simulink model "combined"  (R2023a)
settings: Solver=FixedStepAuto  StartTime=0.0  StopTime=30  RelTol=1e-3
values from neighbouring files (symbols this model uses):
  vehicle_data = getVehicleDataStruct()    [main.m]
libraries: autolibshared x4
settings Model: Creator=ashkan  LastModifiedBy=ashkan
settings OptimizationCC: ReuseModelBlockBuffer=off

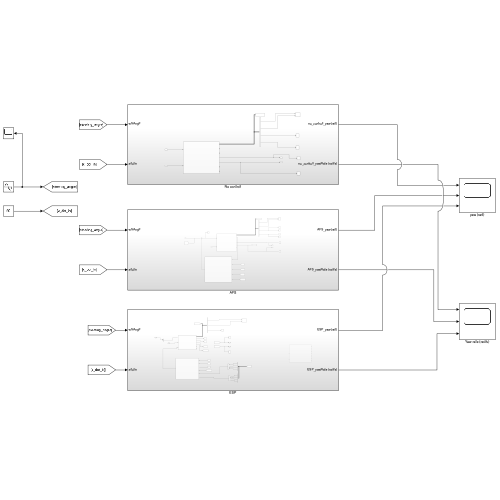
[thumbnail: Simulink's stored preview of the top-level diagram]
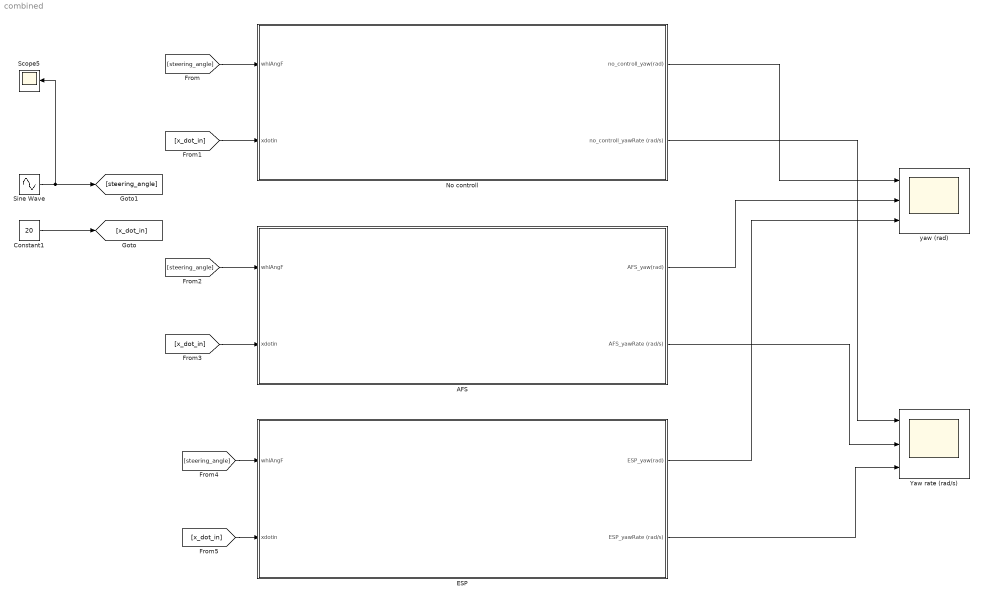
== system combined ==
  AFS : Subsystem
  Constant1 : Constant  Value=20
  ESP : Subsystem
  No controll : Subsystem
  Scope5 : Scope
  Sine Wave : Sin  Amplitude=2  Frequency=0.5  SampleTime=0
  Yaw rate (rad/s) : Scope  NumInputPorts=3
  yaw (rad) : Scope  NumInputPorts=3
  wires:
  Sine Wave/1 -> [steering_angle], Scope5/1
  Constant1/1 -> [x_dot_in]
  [steering_angle] -> No controll/1(whlAngF)
  [x_dot_in] -> No controll/2(xdotin)
  [steering_angle] -> AFS/1(whlAngF)
  [x_dot_in] -> AFS/2(xdotin)
  [steering_angle] -> ESP/1(whlAngF)
  [x_dot_in] -> ESP/2(xdotin)
  No controll/1(no_controll_yaw(rad)) -> yaw (rad)/1
  AFS/1(AFS_yaw(rad)) -> yaw (rad)/2
  ESP/1(ESP_yaw(rad)) -> yaw (rad)/3
  No controll/2(no_controll_yawRate (rad/s)) -> Yaw rate (rad/s)/1
  AFS/2(AFS_yawRate (rad/s)) -> Yaw rate (rad/s)/2
  ESP/2(ESP_yawRate (rad/s)) -> Yaw rate (rad/s)/3

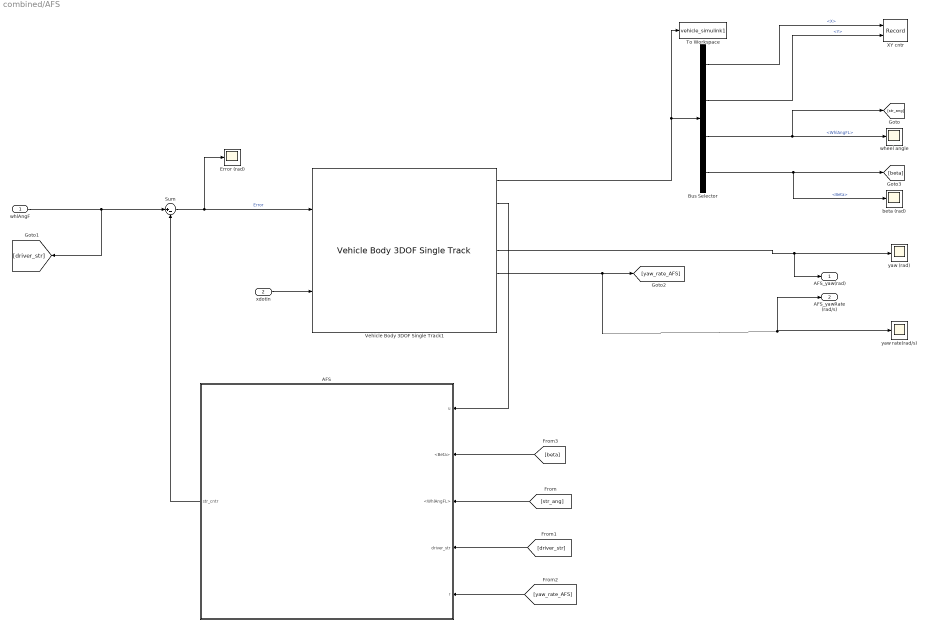
== system combined/AFS ==
  whlAngF : Inport
  xdotin : Inport  Port=2
  AFS : Subsystem
  Bus Selector : BusSelector  OutputSignals=InertFrm.Cg.Disp.X,InertFrm.Cg.Disp.Y,BdyFrm.FrntAxl.Steer.WhlAngFL,BdyFrm.Cg.Ang.Beta
  Error (rad) : Scope
  Sum : Sum  Inputs=|+-
  To Workspace : ToWorkspace  VariableName=vehicle_simulink1  SaveFormat=Timeseries  SampleTime=-1
  Vehicle Body 3DOF Single Track1 : autolibshared/Vehicle Body 3DOF Single Track  trackMode=Single (bicycle)  inputMode=External longitudinal velocity  frontSteerMode=on  rearSteerMode=off  windMode=off  muMode=off  extFMode=off  extMMode=off  htchFMode=off  htchMMode=off  extXo=off  extpsio=off  extxdoto=off  extro=off  extYo=off  extTamb=off  extydoto=off  aMode=2  NF=2  NR=2  m=vehicle_data.vehicle.m  a=vehicle_data.vehicle.Lf  b=vehicle_data.vehicle.Lr  h=vehicle_data.vehicle.hGs  dh=1  hh=0.2  X_o=0  xdot_o=0  CalphaMode=off  sigmaMode=on  d=0  hl=0  w=[1.4,1.4]  Cy_f=vehicle_data.front_suspension.Ks_f  Cy_r=vehicle_data.rear_suspension.Ks_r  sigma_f=.1  sigma_r=.1  alpha_f_brk=[-.1 .1]  Cy_f_data=[-9e3 9e3]  alpha_r_brk=[-.1 .1]  Cy_r_data=[-9e3 9e3]  Y_o=0  ydot_o=0  Izz=vehicle_data.vehicle.i_zz  psi_o=0  r_o=0  Af=2  Cd=.3  Cl=.1  Cpm=.1  beta_w=[0 0.01:0.01:0.3]  Cs=[0 0.01:0.01:0.3]  Cym=[0 1e-6:0.01:0.3]  Pabs=101325  Tair=273  g=9.81  mu=1  xdot_tol=.01  Fznom=5000  Fxtire_sat=7e4  Fytire_sat=7e4  longOff=0  latOff=0  vertOff=0  wrapAng=off
  XY cntr : Record  FileSettingsInternal="{\"entries\":[{\"content\":{\"excelSettings\":{\"content\":{},\"type\":\"Streamout.ExcelSettings\"}},\"type\":\"Streamout.FileSettingStorage\",\"uuid\":\"\"}],\"packageUris\":[\"http:\\/\\/schema.mathworks.com\\/mf0\\/streamout_blocks\\/R2020a\"],\"version\":\"1.0\"}"  Layout=[1 1]  SignalsInternal="{\"entries\":[{\"content\":{\"signals\":[{\"content\":{\"blockPath\":[],\"dimensions\":[1],\"domain\":\"\",\"lineColor\":\"#77ac30\",\"port\":1,\"sid\":[\"\"],\"signalID\":275,\"signalName\":\"<X>\"},\"type\":\"RecordBlkView.Signal\",\"uuid\":\"\"},{\"content\":{\"blockPath\":[],\"dimensions\":[1],\"domain\":\"\",\"lineColor\":\"#4dbeee\",\"port\":2,\"sid\":[\"\"],\"signalID\":279,\"signalName\":\"<Y>\"},\"type\":\"RecordBlkView.Signal\",\"uuid\":\"\"}]},\"type\":\"RecordBlkView.InputSignals\",\"uuid\":\"\"}],\"packageUris\":[\"http:\\/\\/schema.mathworks.com\\/mf0\\/streamout_blocks\\/R2020a\"],\"version\":\"1.0\"}"  VisualizationBindings="{\"xyplotplugin\":{\"info\":[{\"series\":[],\"subplotID\":1}]}}"  CompatibilityTag=XY
  beta (rad) : Scope
  wheel angle : Scope
  yaw (rad) : Scope
  yaw rate(rad/s) : Scope
  AFS_yaw(rad) : Outport
  AFS_yawRate (rad/s) : Outport  Port=2
  wires:
  whlAngF/1 -> [driver_str], Sum/1
  Sum/1 -> Error (rad)/1, Vehicle Body 3DOF Single Track1/1  "Error"
  [yaw_rate_AFS] -> AFS/5(r)
  Bus Selector/3 -> [str_ang], wheel angle/1  "<WhlAngFL>"
  Bus Selector/2 -> XY cntr/2  "<Y>"
  Vehicle Body 3DOF Single Track1/1 -> To Workspace/1, Bus Selector/1
  [beta] -> AFS/2(<Beta>)
  Bus Selector/1 -> XY cntr/1  "<X>"
  Bus Selector/4 -> [beta], beta (rad)/1  "<Beta>"
  AFS/1(str_cntr) -> Sum/2
  Vehicle Body 3DOF Single Track1/2 -> AFS/1(u)
  xdotin/1 -> Vehicle Body 3DOF Single Track1/2
  Vehicle Body 3DOF Single Track1/5 -> [yaw_rate_AFS], AFS_yawRate (rad/s)/1, yaw rate(rad/s)/1
  Vehicle Body 3DOF Single Track1/4 -> AFS_yaw(rad)/1, yaw (rad)/1
  [str_ang] -> AFS/3(<WhlAngFL>)
  [driver_str] -> AFS/4(driver_str)

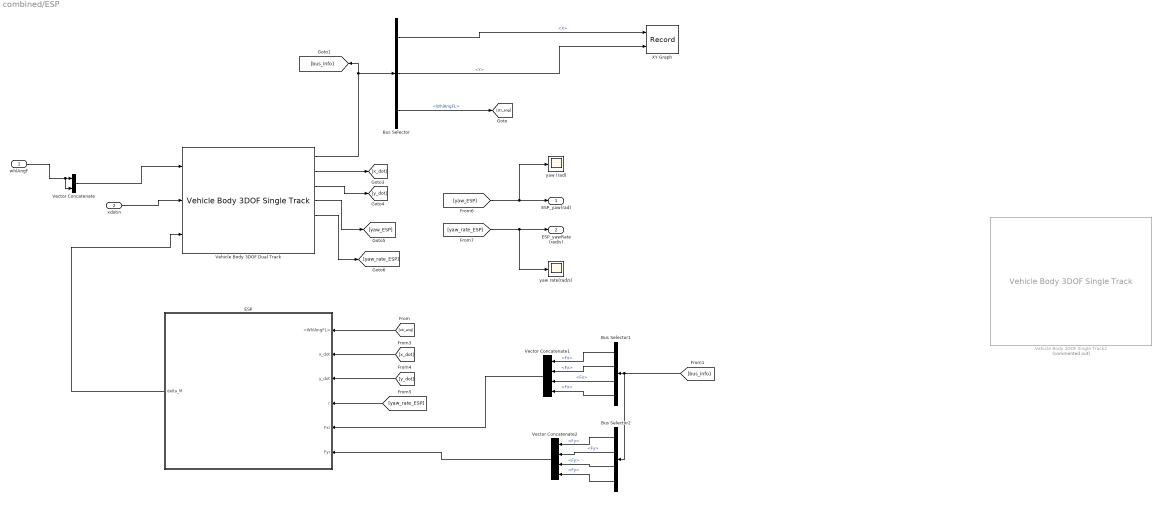
== system combined/ESP ==
  whlAngF : Inport
  xdotin : Inport  Port=2
  Bus Selector : BusSelector  OutputSignals=InertFrm.Cg.Disp.X,InertFrm.Cg.Disp.Y,BdyFrm.FrntAxl.Steer.WhlAngFL
  Bus Selector1 : BusSelector  OutputSignals=BdyFrm.Forces.FrntAxl.Lft.Fx,BdyFrm.Forces.RearAxl.Rght.Fx,BdyFrm.Forces.RearAxl.Lft.Fx,BdyFrm.Forces.FrntAxl.Rght.Fx
  Bus Selector2 : BusSelector  OutputSignals=BdyFrm.Forces.FrntAxl.Lft.Fy,BdyFrm.Forces.FrntAxl.Rght.Fy,BdyFrm.Forces.RearAxl.Lft.Fy,BdyFrm.Forces.RearAxl.Rght.Fy
  ESP : Subsystem
  Vector Concatenate : Concatenate
  Vector Concatenate1 : Concatenate  NumInputs=4
  Vector Concatenate2 : Concatenate  NumInputs=4
  Vehicle Body 3DOF Dual Track : autolibshared/Vehicle Body 3DOF Single Track  trackMode=Dual  inputMode=External longitudinal velocity  frontSteerMode=on  rearSteerMode=off  windMode=off  muMode=off  extFMode=off  extMMode=on  htchFMode=off  htchMMode=off  extXo=off  extpsio=off  extxdoto=off  extro=off  extYo=off  extTamb=off  extydoto=off  aMode=2  NF=2  NR=2  m=2000  a=1.4  b=1.6  h=0.35  dh=1  hh=0.2  X_o=0  xdot_o=0  CalphaMode=off  sigmaMode=on  d=0  hl=0  w=[1.4,1.4]  Cy_f=12e3  Cy_r=11e3  sigma_f=.1  sigma_r=.1  alpha_f_brk=[-.1 .1]  Cy_f_data=[-9e3 9e3]  alpha_r_brk=[-.1 .1]  Cy_r_data=[-9e3 9e3]  Y_o=0  ydot_o=0  Izz=4000  psi_o=0  r_o=0  Af=2  Cd=.3  Cl=.1  Cpm=.1  beta_w=[0 0.01:0.01:0.3]  Cs=[0:0.03:0.9]  Cym=[0 1e-6:0.01:0.3]  Pabs=101325  Tair=273  g=9.81  mu=1  xdot_tol=.01  Fznom=5000  Fxtire_sat=7e4  Fytire_sat=7e4  longOff=0  latOff=0  vertOff=0  wrapAng=off
      settings: LibrarySourceBlock=vehdynlibeom/Vehicle Body 3DOF Dual Track
  Vehicle Body 3DOF Single Track2 : autolibshared/Vehicle Body 3DOF Single Track  Commented=on  trackMode=Dual  inputMode=External longitudinal velocity  frontSteerMode=on  rearSteerMode=off  windMode=off  muMode=off  extFMode=off  extMMode=on  htchFMode=off  htchMMode=off  extXo=off  extpsio=off  extxdoto=off  extro=off  extYo=off  extTamb=off  extydoto=off  aMode=2  NF=2  NR=2  m=vehicle_data.vehicle.m  a=vehicle_data.vehicle.Lf  b=vehicle_data.vehicle.Lr  h=vehicle_data.vehicle.hGs  dh=1  hh=0.2  X_o=0  xdot_o=0  CalphaMode=off  sigmaMode=on  d=0  hl=0  w=[vehicle_data.vehicle.Wf,vehicle_data.vehicle.Wr]  Cy_f=vehicle_data.front_suspension.Ks_f  Cy_r=vehicle_data.rear_suspension.Ks_r  sigma_f=vehicle_data.vehicle.lx  sigma_r=vehicle_data.vehicle.ly  alpha_f_brk=[-.1 .1]  Cy_f_data=[-9e3 9e3]  alpha_r_brk=[-.1 .1]  Cy_r_data=[-9e3 9e3]  Y_o=0  ydot_o=0  Izz=vehicle_data.vehicle.i_zz  psi_o=0  r_o=0  Af=2  Cd=vehicle_data.aerodynamics.CAx  Cl=vehicle_data.aerodynamics.CAzf  Cpm=.1  beta_w=[0 0.01:0.01:0.3]  Cs=[0 0.01:0.01:0.3]  Cym=[0 1e-6:0.01:0.3]  Pabs=101325  Tair=273  g=9.81  mu=0.9  xdot_tol=.02  Fznom=5000  Fxtire_sat=7e4  Fytire_sat=7e4  longOff=0  latOff=0  vertOff=0  wrapAng=off
  XY Graph : Record  FileSettingsInternal="{\"entries\":[{\"content\":{\"excelSettings\":{\"content\":{},\"type\":\"Streamout.ExcelSettings\"}},\"type\":\"Streamout.FileSettingStorage\",\"uuid\":\"\"}],\"packageUris\":[\"http:\\/\\/schema.mathworks.com\\/mf0\\/streamout_blocks\\/R2020a\"],\"version\":\"1.0\"}"  Layout=[1 1]  SignalsInternal="{\"entries\":[{\"content\":{\"signals\":[{\"content\":{\"blockPath\":[],\"dimensions\":[1],\"domain\":\"\",\"lineColor\":\"#d95319\",\"plots\":[1],\"port\":1,\"sid\":[\"\"],\"signalID\":1078,\"signalName\":\"<X>\"},\"type\":\"RecordBlkView.Signal\",\"uuid\":\"\"},{\"content\":{\"blockPath\":[],\"dimensions\":[1],\"domain\":\"\",\"lineColor\":\"#edb120\",\"plots\":[1],\"port\":2,\"sid\":[\"\"],\"signalID\":1082,\"signalName\":\"<Y>\"},\"type\":\"RecordBlkView.Signal\",\"uuid\":\"\"}]},\"type\":\"RecordBlkView.InputSignals\",\"uuid\":\"\"}],\"packageUris\":[\"http:\\/\\/schema.mathworks.com\\/mf0\\/streamout_blocks\\/R2020a\"],\"version\":\"1.0\"}"  VisualizationBindings="{\"xyplotplugin\":{\"info\":[{\"series\":[{\"bindingParametersList\":[{\"parameter\":\"X-Axis\",\"signalID\":1078,\"signalName\":\"<X>\"},{\"parameter\":\"Y-Axis\",\"signalID\":1082,\"signalName\":\"<Y>\"}],\"seriesID\":10530}],\"subplotID\":1}]}}"  CompatibilityTag=XY
  yaw (rad) : Scope
  yaw rate(rad/s) : Scope
  ESP_yaw(rad) : Outport
  ESP_yawRate (rad/s) : Outport  Port=2
  wires:
  [yaw_rate_ESP] -> ESP_yawRate (rad/s)/1, yaw rate(rad/s)/1
  Vehicle Body 3DOF Dual Track/3 -> [y_dot]
  [yaw_ESP] -> ESP_yaw(rad)/1, yaw (rad)/1
  [x_dot] -> ESP/2(x_dot)
  Vehicle Body 3DOF Dual Track/5 -> [yaw_rate_ESP]
  [y_dot] -> ESP/3(y_dot)
  Bus Selector/3 -> [str_ang]  "<WhlAngFL>"
  Vehicle Body 3DOF Dual Track/4 -> [yaw_ESP]
  Vehicle Body 3DOF Dual Track/2 -> [x_dot]
  [yaw_rate_ESP] -> ESP/4(r)
  Bus Selector/2 -> XY Graph/2  "<Y>"
  [str_ang] -> ESP/1(<WhlAngFL>)
  Bus Selector/1 -> XY Graph/1  "<X>"
  Vehicle Body 3DOF Dual Track/1 -> [bus_info], Bus Selector/1
  xdotin/1 -> Vehicle Body 3DOF Dual Track/2
  whlAngF/1 -> Vector Concatenate/2, Vector Concatenate/1
  Vector Concatenate/1 -> Vehicle Body 3DOF Dual Track/1
  [bus_info] -> Bus Selector2/1, Bus Selector1/1
  Bus Selector1/1 -> Vector Concatenate1/1  "<Fx>"
  Bus Selector1/2 -> Vector Concatenate1/2  "<Fx>"
  Bus Selector1/3 -> Vector Concatenate1/3  "<Fx>"
  Bus Selector1/4 -> Vector Concatenate1/4  "<Fx>"
  Bus Selector2/1 -> Vector Concatenate2/1  "<Fy>"
  Bus Selector2/2 -> Vector Concatenate2/2  "<Fy>"
  Bus Selector2/3 -> Vector Concatenate2/3  "<Fy>"
  Bus Selector2/4 -> Vector Concatenate2/4  "<Fy>"
  Vector Concatenate2/1 -> ESP/6(Fyi)
  Vector Concatenate1/1 -> ESP/5(Fxi)
  ESP/1(delta_M) -> Vehicle Body 3DOF Dual Track/3

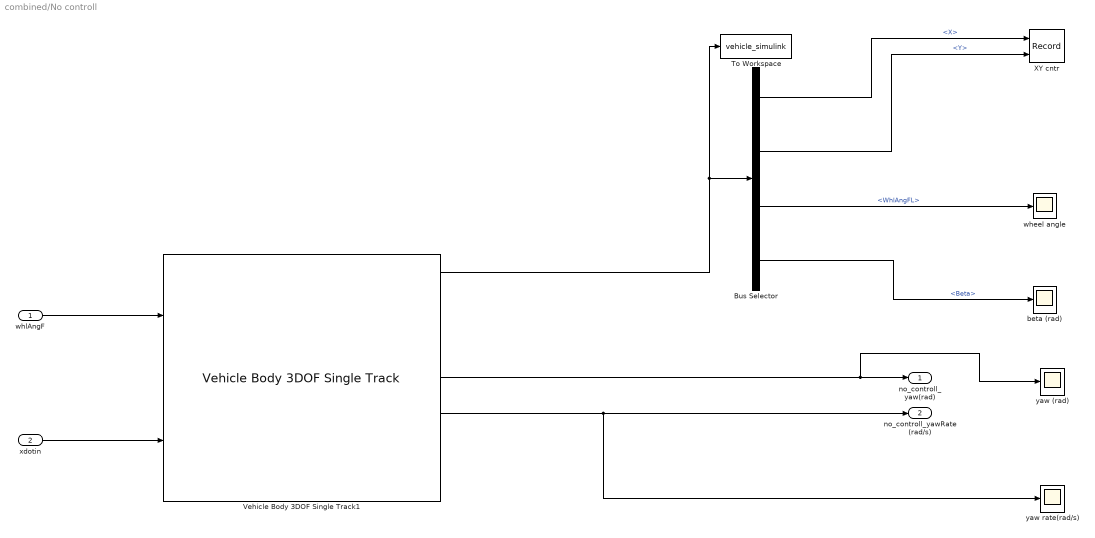
== system combined/No controll ==
  whlAngF : Inport
  xdotin : Inport  Port=2
  Bus Selector : BusSelector  OutputSignals=InertFrm.Cg.Disp.X,InertFrm.Cg.Disp.Y,BdyFrm.FrntAxl.Steer.WhlAngFL,BdyFrm.Cg.Ang.Beta
  To Workspace : ToWorkspace  VariableName=vehicle_simulink  SaveFormat=Timeseries  SampleTime=-1
  Vehicle Body 3DOF Single Track1 : autolibshared/Vehicle Body 3DOF Single Track  trackMode=Single (bicycle)  inputMode=External longitudinal velocity  frontSteerMode=on  rearSteerMode=off  windMode=off  muMode=off  extFMode=off  extMMode=off  htchFMode=off  htchMMode=off  extXo=off  extpsio=off  extxdoto=off  extro=off  extYo=off  extTamb=off  extydoto=off  aMode=2  NF=2  NR=2  m=vehicle_data.vehicle.m  a=vehicle_data.vehicle.Lf  b=vehicle_data.vehicle.Lr  h=vehicle_data.vehicle.hGs  dh=1  hh=0.2  X_o=0  xdot_o=0  CalphaMode=off  sigmaMode=on  d=0  hl=0  w=[1.4,1.4]  Cy_f=vehicle_data.front_suspension.Ks_f  Cy_r=vehicle_data.rear_suspension.Ks_r  sigma_f=.1  sigma_r=.1  alpha_f_brk=[-.1 .1]  Cy_f_data=[-9e3 9e3]  alpha_r_brk=[-.1 .1]  Cy_r_data=[-9e3 9e3]  Y_o=0  ydot_o=0  Izz=vehicle_data.vehicle.i_zz  psi_o=0  r_o=0  Af=2  Cd=.3  Cl=.1  Cpm=.1  beta_w=[0 0.01:0.01:0.3]  Cs=[0 0.01:0.01:0.3]  Cym=[0 1e-6:0.01:0.3]  Pabs=101325  Tair=273  g=9.81  mu=1  xdot_tol=.01  Fznom=5000  Fxtire_sat=7e4  Fytire_sat=7e4  longOff=0  latOff=0  vertOff=0  wrapAng=off
  XY cntr : Record  FileSettingsInternal="{\"entries\":[{\"content\":{\"excelSettings\":{\"content\":{},\"type\":\"Streamout.ExcelSettings\"}},\"type\":\"Streamout.FileSettingStorage\",\"uuid\":\"\"}],\"packageUris\":[\"http:\\/\\/schema.mathworks.com\\/mf0\\/streamout_blocks\\/R2020a\"],\"version\":\"1.0\"}"  Layout=[1 1]  SignalsInternal="{\"entries\":[{\"content\":{\"signals\":[{\"content\":{\"blockPath\":[],\"dimensions\":[1],\"domain\":\"\",\"lineColor\":\"#22b573\",\"port\":1,\"sid\":[\"\"],\"signalID\":1099,\"signalName\":\"<X>\"},\"type\":\"RecordBlkView.Signal\",\"uuid\":\"\"},{\"content\":{\"blockPath\":[],\"dimensions\":[1],\"domain\":\"\",\"lineColor\":\"#0072bd\",\"port\":2,\"sid\":[\"\"],\"signalID\":1103,\"signalName\":\"<Y>\"},\"type\":\"RecordBlkView.Signal\",\"uuid\":\"\"}]},\"type\":\"RecordBlkView.InputSignals\",\"uuid\":\"\"}],\"packageUris\":[\"http:\\/\\/schema.mathworks.com\\/mf0\\/streamout_blocks\\/R2020a\"],\"version\":\"1.0\"}"  VisualizationBindings="{\"xyplotplugin\":{\"info\":[{\"series\":[],\"subplotID\":1}]}}"  CompatibilityTag=XY
  beta (rad) : Scope
  wheel angle : Scope
  yaw (rad) : Scope
  yaw rate(rad/s) : Scope
  no_controll_yaw(rad) : Outport
  no_controll_yawRate (rad/s) : Outport  Port=2
  wires:
  xdotin/1 -> Vehicle Body 3DOF Single Track1/2
  Vehicle Body 3DOF Single Track1/1 -> To Workspace/1, Bus Selector/1
  Bus Selector/2 -> XY cntr/2  "<Y>"
  Vehicle Body 3DOF Single Track1/5 -> yaw rate(rad/s)/1, no_controll_yawRate (rad/s)/1
  Bus Selector/1 -> XY cntr/1  "<X>"
  whlAngF/1 -> Vehicle Body 3DOF Single Track1/1
  Bus Selector/3 -> wheel angle/1  "<WhlAngFL>"
  Bus Selector/4 -> beta (rad)/1  "<Beta>"
  Vehicle Body 3DOF Single Track1/4 -> yaw (rad)/1, no_controll_yaw(rad)/1

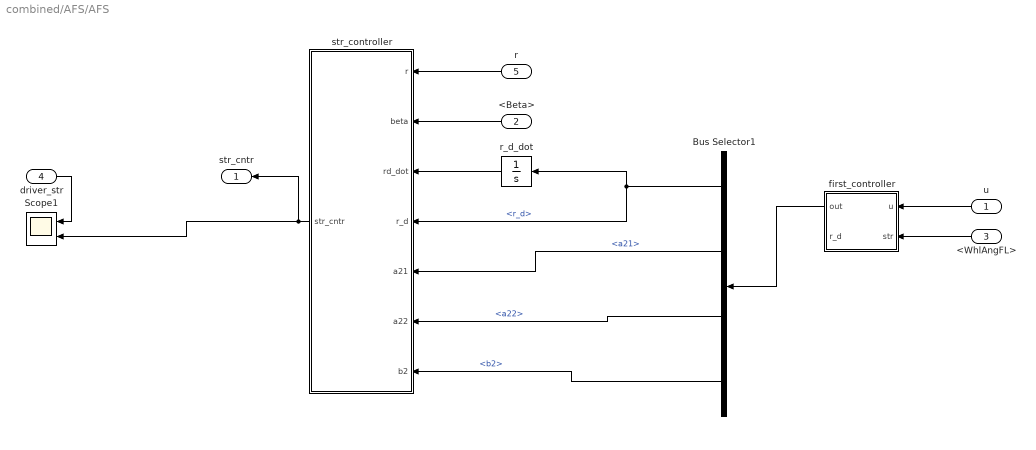
== system combined/AFS/AFS ==
  u : Inport
  <Beta> : Inport  Port=2
  <WhlAngFL> : Inport  Port=3
  driver_str : Inport  Port=4
  r : Inport  Port=5
  Bus Selector1 : BusSelector  OutputSignals=r_d,a21,a22,b2
  Scope1 : Scope  NumInputPorts=2
  first_controller : MATLAB Function  TreatAsAtomicUnit=on
  r_d_dot : Integrator
  str_controller : MATLAB Function  TreatAsAtomicUnit=on
  str_cntr : Outport
  wires:
  driver_str/1 -> Scope1/1
  <Beta>/1 -> str_controller/2(beta)
  r/1 -> str_controller/1(r)
  first_controller/1(out) -> Bus Selector1/1
  <WhlAngFL>/1 -> first_controller/2(str)
  u/1 -> first_controller/1(u)
  Bus Selector1/2 -> str_controller/5(a21)  "<a21>"
  Bus Selector1/3 -> str_controller/6(a22)  "<a22>"
  str_controller/1(str_cntr) -> Scope1/2, str_cntr/1
  r_d_dot/1 -> str_controller/3(rd_dot)
  Bus Selector1/1 -> str_controller/4(r_d), r_d_dot/1  "<r_d>"
  Bus Selector1/4 -> str_controller/7(b2)  "<b2>"

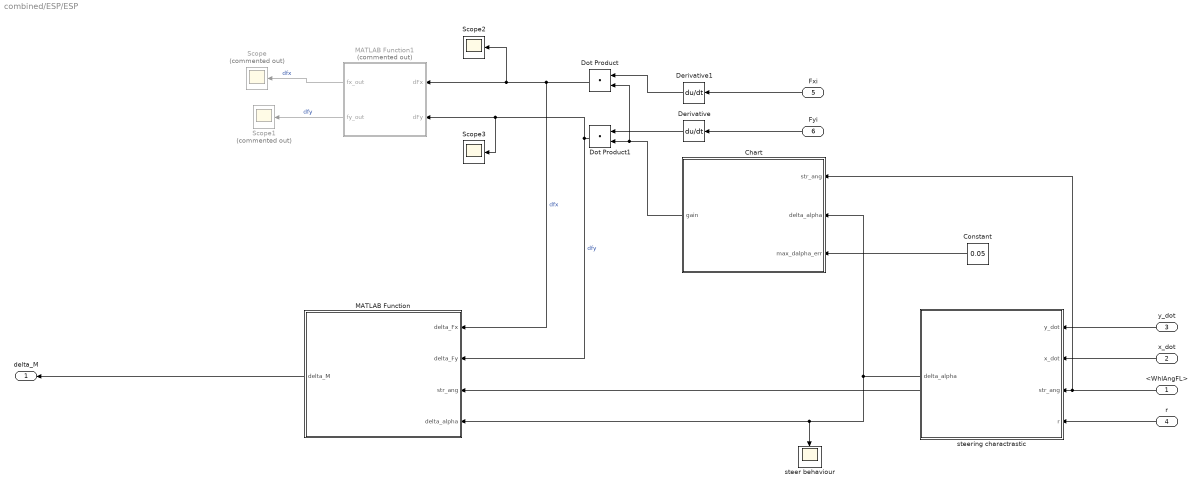
== system combined/ESP/ESP ==
  <WhlAngFL> : Inport
  x_dot : Inport  Port=2
  y_dot : Inport  Port=3
  r : Inport  Port=4
  Fxi : Inport  Port=5
  Fyi : Inport  Port=6
  Chart : Stateflow chart  TreatAsAtomicUnit=on
  Constant : Constant  Value=0.05
  Derivative : Derivative
  Derivative1 : Derivative
  Dot Product : DotProduct  OutDataTypeStr=Inherit: Inherit via internal rule
  Dot Product1 : DotProduct  OutDataTypeStr=Inherit: Inherit via internal rule
  MATLAB Function : MATLAB Function  TreatAsAtomicUnit=on
  MATLAB Function1 : MATLAB Function  Commented=on  TreatAsAtomicUnit=on
  Scope : Scope  Commented=on
  Scope1 : Scope  Commented=on
  Scope2 : Scope
  Scope3 : Scope
  steer behaviour : Scope
  steering charactrastic : MATLAB Function  TreatAsAtomicUnit=on
  delta_M : Outport
  wires:
  x_dot/1 -> steering charactrastic/2(x_dot)
  steering charactrastic/1(delta_alpha) -> Chart/2(delta_alpha), MATLAB Function/4(delta_alpha), steer behaviour/1
  r/1 -> steering charactrastic/4(r)
  y_dot/1 -> steering charactrastic/1(y_dot)
  <WhlAngFL>/1 -> MATLAB Function/3(str_ang), steering charactrastic/3(str_ang), Chart/1(str_ang)
  MATLAB Function/1(delta_M) -> delta_M/1
  Constant/1 -> Chart/3(max_dalpha_err)
  Chart/1(gain) -> Dot Product1/2, Dot Product/2
  Fxi/1 -> Derivative1/1
  Fyi/1 -> Derivative/1
  Derivative1/1 -> Dot Product/1
  Dot Product/1 -> MATLAB Function/1(delta_Fx), Scope2/1, MATLAB Function1/1(dFx)  "dfx"
  Derivative/1 -> Dot Product1/1
  Dot Product1/1 -> MATLAB Function/2(delta_Fy), Scope3/1, MATLAB Function1/2(dFy)  "dfy"
  MATLAB Function1/1(fx_out) -> Scope/1  "dfx"
  MATLAB Function1/2(fy_out) -> Scope1/1  "dfy"

== matlab function combined/ESP/ESP/MATLAB Function1 ==
  data: dFx input; fx_out output; dFy input; fy_out output
function [fx_out , fy_out] = whl_select(dFx , dFy)
    
    s = length(dFx);
    
    for i=1:s
        if dFy(i) > 0 
            fy_out = dFy(i);
            fx_out = dFx(i);
        else
            fy_out = 0;
            fx_out = 0;

    end

end

== stateflow chart combined/ESP/ESP/Chart ==
  state ESP_ON
    state FRONT_WHEEL
      state FRONT_LEFT
        gain = [1 0 0 0];
      state FRONT_RIGHT
        gain = [0 1 0 0] ;
      (junction 36) -> FRONT_LEFT [order 2] : [str_ang <0]
      (junction 36) -> FRONT_RIGHT [order 1] : [str_ang >     0]
      FRONT_RIGHT -> (junction 36)
      FRONT_LEFT -> (junction 36)
    state REAR_WHEEL
      state REAR_LEFT
        gain = [0 0 1 0];
      state REAR_RIGHT
        gain = [0 0 0 1];
      (junction 38) -> REAR_LEFT [order 1] : [str_ang > 0]
      (junction 38) -> REAR_RIGHT [order 2] : [str_ang < 0]
      REAR_RIGHT -> (junction 38)
      REAR_LEFT -> (junction 38)
    (junction 31) -> (junction 36) [order 1] : [delta_alpha > 0 ]
    FRONT_WHEEL -> (junction 31)
    REAR_WHEEL -> (junction 31)
    (junction 31) -> (junction 38) [order 2] : [delta_alpha < 0]
  state ESP_OFF
    gain = [0 0 0 0]   ;
  (default) -> ESP_OFF
  ESP_OFF -> (junction 31) : [ abs(delta_alpha) > max_dalpha_err + 0.01   ]
  ESP_ON -> ESP_OFF : [abs(delta_alpha  ) < max_dalpha_err - 0.01]
  data: str_ang input; delta_alpha input; max_dalpha_err input; gain output

== matlab function combined/AFS/AFS/str_controller ==
  data: r input; beta input; rd_dot input; r_d input; a21 input; str_cntr output; a22 input; b2 input; vehicle_data parameter
function str_cntr = str_controller(r, beta , rd_dot , r_d , a21 , a22 , b2, vehicle_data)

%    lambda = AFS.lambda;
    s = r - r_d;
    lambda = vehicle_data.AFS.lambda;
    X      = vehicle_data.AFS.X;
    str_cntr = ((1/b2) * (-a21*beta - a22*r + rd_dot - lambda*(r - r_d))) - sign(s)*X;


end

== matlab function combined/AFS/AFS/first_controller ==
  data: out output Bus: out_rd_bus; u input; str input; vehicle_data parameter; r_d output
function [out, r_d] = r_d(u , str, vehicle_data)


% here is some simplified parameters :)
   m = vehicle_data.vehicle.m;
   a = vehicle_data.vehicle.Lf;
   b = vehicle_data.vehicle.Lr;
   izz = vehicle_data.vehicle.i_zz;
   g = vehicle_data.vehicle.g;
   L = vehicle_data.vehicle.L;
   mu = vehicle_data.AFS.mu;  % --> should come from scenario
   Caf = vehicle_data.front_suspension.Ks_f ;
   Car = vehicle_data.rear_suspension.Ks_r;
   
   
% lets calculate some live parameters!!! _|_
    
   r_up_lim = 0.85 * abs(mu*g / u);
   r_ss = (2*L*Caf*Car*u)/(2*Car*Caf*L^2 - m*u^2*(a*Caf - b*Car)) * str;
   r_d = min(r_ss , r_up_lim)* sign(str);
 
   a11 = (-2*Caf - 2*Car)/(m * u);
   a12 = -1 + (2*Car*b - 2*Caf*a)/(m * u^2);
   a21 = (2*Car*b - 2*Caf*a)/izz;
   a22 = (-2*Caf*a^2 - 2*Car*b^2)/(izz * u);
   b1 = (2*Caf)/(m * u);
   b2 = (2 * Caf * a)/izz;

% outputs
   out.a11 = a11;
   out.a21 = a21;
   out.a12 = a12;
   out.a22 = a22;
   out.b1 = b1;
   out.b2 = b2;
   out.r_d = r_d;

end

== matlab function combined/ESP/ESP/MATLAB Function ==
  data: delta_Fx input; delta_M output; delta_Fy input; str_ang input; delta_alpha input; vehicle_data parameter
function delta_M   = yaw_moment_diff(delta_Fx , delta_Fy ,  str_ang , delta_alpha , vehicle_data)

    a = vehicle_data.vehicle.Lf;
    b = vehicle_data.vehicle.Lr;
    L = vehicle_data.vehicle.L;
    Tw = vehicle_data.vehicle.Wf;

    if delta_alpha > 0      % over steering

    
        delta_Mz = (delta_Fx*(0.5*Tw*cos(str_ang) + a*sin(str_ang))) - (delta_Fy * (a*cos(str_ang) - 0.5*Tw*sin(str_ang)));

        
    elseif delta_alpha < 0  % under steering

        
        delta_Mz = (delta_Fx * 0.5*Tw) - (delta_Fy * b);

    else    % natural steering
        delta_Mz = 0;

    end

    delta_Mx = 0;

    delta_My = 0;

    delta_M = [delta_Mx , delta_My , delta_Mz];

end

== matlab function combined/ESP/ESP/steering charactrastic ==
  data: y_dot input; x_dot input; delta_alpha output; str_ang input; r input; vehicle_data parameter
function delta_alpha = steer_char(y_dot , x_dot , str_ang , r , vehicle_data)

    a = vehicle_data.vehicle.Lf;
    b = vehicle_data.vehicle.Lr;

    alpha_f = str_ang - atan((y_dot + a*r)/(x_dot));
    alpha_r = -atan((y_dot - b*r)/(x_dot));

    delta_alpha = alpha_r - alpha_f;

end
